simulink model "PolePlaceHeliGain"  (R2021a)
settings: Solver=VariableStepAuto  StartTime=0.0  StopTime=10.0  MaxStep=1e-3  RelTol=1e-3
values from neighbouring files (symbols this model uses):
  A = [0 0 1 0 ... (first row only)    [HeliControlGain.m]    (also in HeliControlHinf.m; HeliControlInteger.m; HeliControlLQG.m; HeliControlLQRgain.m)
  B = [0 0 ... (first row only)    [HeliControlGain.m]    (also in HeliControlHinf.m; HeliControlInteger.m; HeliControlLQG.m; HeliControlLQRgain.m)
  C = [1 0 0 0 ... (first row only)    [HeliControlGain.m]    (also in HeliControlHinf.m; HeliControlInteger.m; HeliControlLQG.m; HeliControlLQRgain.m)
  D = zeros(2,2)    [HeliControlGain.m]    (also in HeliControlHinf.m; HeliControlInteger.m; HeliControlLQG.m; HeliControlLQRgain.m)
  G = Gbar\I    [HeliControlGain.m]    (also in HeliControlHinf.m = ss(A,B,C,D); HeliControlLQRgain.m)
  K = place(A,B,p)    [HeliControlGain.m]    (also in HeliControlInteger.m = place(Ag,Bg,p); HeliControlIntegerObsv.m = place(Ag,Bg,p); HeliControlLQG.m = lqr(Ag,Bg,Q,R); HeliControlLQRgain.m = lqr(sysHeli,Q,R))
settings Model: Creator=Ciro  LastModifiedBy=Ciro

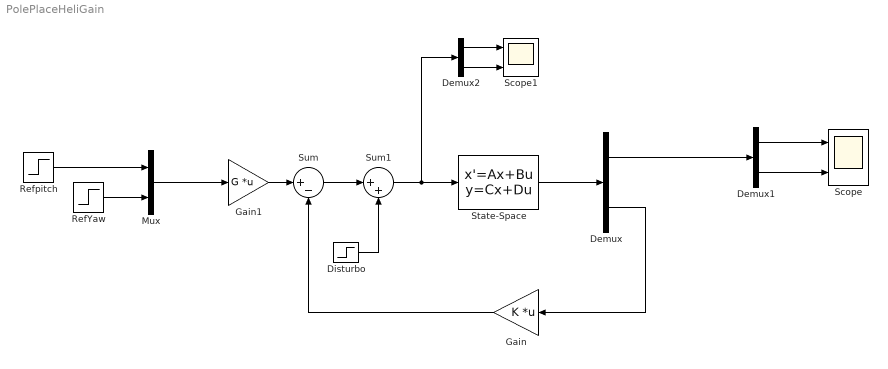
== system PolePlaceHeliGain ==
  Demux : Demux  Outputs=[2 4]
  Demux1 : Demux  Outputs=2
  Demux2 : Demux  Outputs=2
  Disturbo : Step  Time=6  After=0  SampleTime=0
  Gain : Gain  Gain=K  Multiplication=Matrix(K*u)
  Gain1 : Gain  Gain=G  Multiplication=Matrix(K*u)
  Mux : Mux  Inputs=2
  RefYaw : Step  After=0.3  SampleTime=0
  Refpitch : Step  After=0.3  SampleTime=0
  Scope : Scope  NumInputPorts=2
  Scope1 : Scope  NumInputPorts=2
  State-Space : StateSpace  A=A  B=B  C=[C;eye(4)]  D=[D;zeros(4,2)]  InitialCondition=[0;0;0;0]
  Sum : Sum  Inputs=|+-
  Sum1 : Sum  Inputs=|++
  wires:
  Demux2/2 -> Scope1/2
  Sum/1 -> Sum1/1
  Demux/2 -> Gain/1
  Sum1/1 -> State-Space/1, Demux2/1
  Gain1/1 -> Sum/1
  Demux1/1 -> Scope/1
  Demux/1 -> Demux1/1
  Demux2/1 -> Scope1/1
  RefYaw/1 -> Mux/2
  Demux1/2 -> Scope/2
  State-Space/1 -> Demux/1
  Gain/1 -> Sum/2
  Refpitch/1 -> Mux/1
  Mux/1 -> Gain1/1
  Disturbo/1 -> Sum1/2
